simulink model "Week2_problem4"  (R2020b)
settings: Solver=VariableStepAuto  StartTime=0.0  StopTime=10.0  RelTol=1e-3
settings Model: DataDictionary=motor_dict.sldd  Creator=omkar  LastModifiedBy=omkar

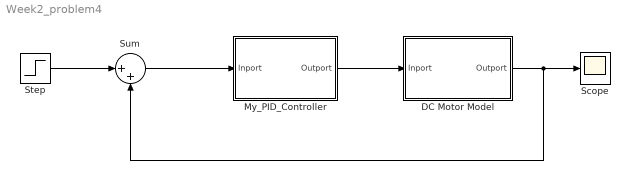
== system Week2_problem4 ==
  DC Motor Model : Subsystem  mask{L=2.75E-6, J=3.2284E-6, R=4, b=3.5077E-6, K=0.0274}
      mask Display: disp('DC Motor')
  My_PID_Controller : Subsystem  mask{Kp=-23.0264121536819, Ki=-759.153316198618, Kd=-0.168220548295185}
      mask Display: disp('P.I.D Controller')
  Scope : Scope
  Step : Step  Time=0  After=150  SampleTime=0
  Sum : Sum  Inputs=|++
  wires:
  Step/1 -> Sum/1
  DC Motor Model/1(Outport) -> Sum/2, Scope/1
  Sum/1 -> My_PID_Controller/1(Inport)
  My_PID_Controller/1(Outport) -> DC Motor Model/1(Inport)

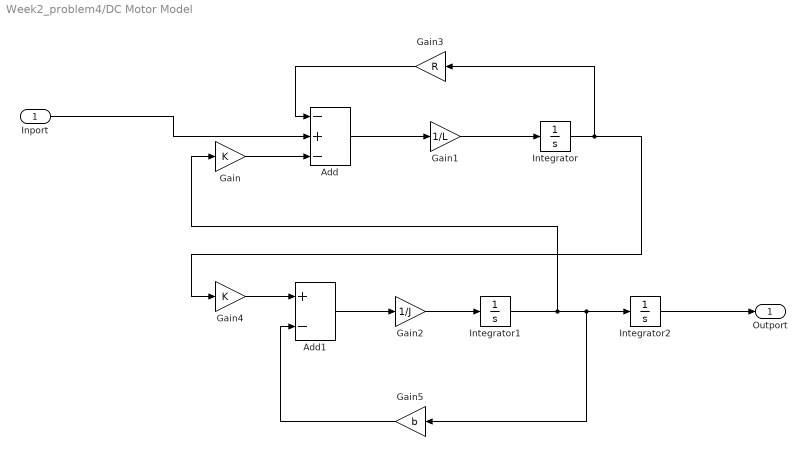
== system Week2_problem4/DC Motor Model ==
  Inport : Inport
  Add : Sum  Inputs=-+-
  Add1 : Sum  Inputs=+-
  Gain : Gain  Gain=K
  Gain1 : Gain  Gain=1/L
  Gain2 : Gain  Gain=1/J
  Gain3 : Gain  Gain=R
  Gain4 : Gain  Gain=K
  Gain5 : Gain  Gain=b
  Integrator : Integrator
  Integrator1 : Integrator
  Integrator2 : Integrator
  Outport : Outport
  wires:
  Gain/1 -> Add/3
  Integrator2/1 -> Outport/1
  Integrator1/1 -> Gain/1, Gain5/1, Integrator2/1
  Gain5/1 -> Add1/2
  Inport/1 -> Add/2
  Gain2/1 -> Integrator1/1
  Gain3/1 -> Add/1
  Integrator/1 -> Gain4/1, Gain3/1
  Add/1 -> Gain1/1
  Gain1/1 -> Integrator/1
  Add1/1 -> Gain2/1
  Gain4/1 -> Add1/1

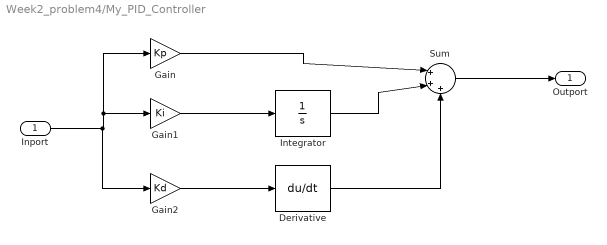
== system Week2_problem4/My_PID_Controller ==
  Inport : Inport
  Derivative : Derivative
  Gain : Gain  Gain=Kp
  Gain1 : Gain  Gain=Ki
  Gain2 : Gain  Gain=Kd
  Integrator : Integrator
  Sum : Sum  Inputs=|+++
  Outport : Outport
  wires:
  Sum/1 -> Outport/1
  Gain2/1 -> Derivative/1
  Gain/1 -> Sum/1
  Derivative/1 -> Sum/3
  Gain1/1 -> Integrator/1
  Integrator/1 -> Sum/2
  Inport/1 -> Gain2/1, Gain1/1, Gain/1
